simulink model "PSK"  (R2021a)
settings: Solver=VariableStepAuto  StartTime=0.0  StopTime=10.0  RelTol=1e-3
settings Model: Creator=Bharat Gunhalkar  LastModifiedBy=Bharat Gunhalkar

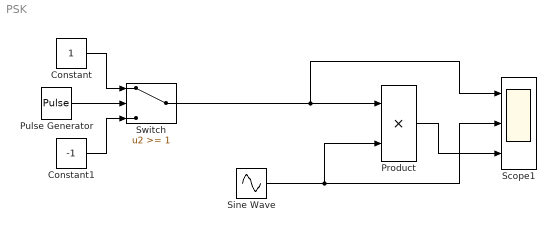
== system PSK ==
  Constant : Constant
  Constant1 : Constant  Value=-1
  Product : Product
  Pulse Generator : DiscretePulseGenerator  PulseType=Time based  PulseWidth=50
  Scope1 : Scope  NumInputPorts=3
  Sine Wave : Sin  Amplitude=14.142  Frequency=2*pi*1000  Phase=90  SampleTime=0
  Switch : Switch  Threshold=1
  wires:
  Pulse Generator/1 -> Switch/2
  Constant1/1 -> Switch/3
  Switch/1 -> Scope1/1, Product/1
  Sine Wave/1 -> Scope1/2, Product/2
  Product/1 -> Scope1/3
  Constant/1 -> Switch/1
